simulink model "inverted_pendulum_without_interpreted_function"  (R2018a)
settings: Solver=VariableStepAuto  StartTime=0.0  StopTime=30  RelTol=1e-3
values from neighbouring files (symbols this model uses):
  A = [0 1 0 0 ... (first row only)    [lqr_d_cartpend.m]
  A_d = sys_d.A    [lqr_d_cartpend.m]
  B = [0; 1/M; 0; s*1/(M*L)]    [lqr_d_cartpend.m]
  B_d = sys_d.B    [lqr_d_cartpend.m]
  C = [1 1 1 1]    [lqr_d_cartpend.m]
  C_d = sys_d.C    [lqr_d_cartpend.m]
  Ts = 0.1    [lqr_d_cartpend.m]
  y0 = [-3; 0; pi + pi/4; 0]    [lqr_d_cartpend.m]
undefined symbols (not defined in the file or in its folder): Kd, Obd
libraries: fl_lib x4, nesl_utility x4, elec_lib x3
settings Model: EnablePacing=on  PacingRate=1000  Creator=USER  LastModifiedBy=USER

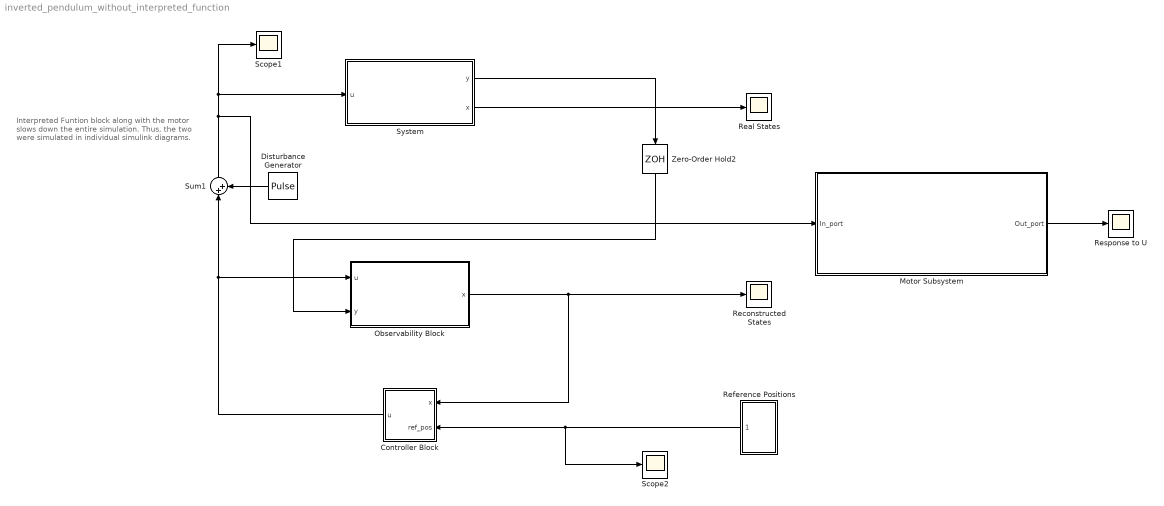
== system inverted_pendulum_without_interpreted_function ==
  note: Interpreted Funtion block along with the motor slows down the entire simulation. Thus, the two were simulated in individual simulink diagrams.
  Controller Block : Subsystem
  Disturbance Generator : DiscretePulseGenerator  PulseType=Time based  Amplitude=20  Period=10  PulseWidth=50  PhaseDelay=10
  Motor Subsystem : Subsystem
  Observability Block : Subsystem
  Real States : Scope
  Reconstructed States : Scope
  Reference Positions : Subsystem
  Response to U : Scope
  Scope1 : Scope
  Scope2 : Scope
  Sum1 : Sum  Inputs=|++
  System : Subsystem
  Zero-Order Hold2 : ZeroOrderHold  SampleTime=Ts
  wires:
  Reference Positions/1(ref_pos) -> Controller Block/2(ref_pos), Scope2/1
  Observability Block/1("x ") -> Reconstructed States/1, Controller Block/1("x ")
  System/1("y ") -> Zero-Order Hold2/1
  Zero-Order Hold2/1 -> Observability Block/2(y)
  System/2("x ") -> Real States/1
  Disturbance Generator/1 -> Sum1/2
  Sum1/1 -> Motor Subsystem/1(In_port), Scope1/1, System/1("u ")
  Motor Subsystem/1(Out_port) -> Response to U/1
  Controller Block/1("u ") -> Sum1/1, Observability Block/1("u ")

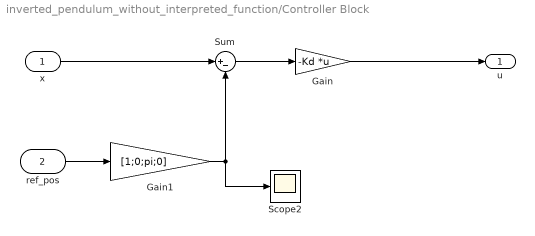
== system inverted_pendulum_without_interpreted_function/Controller Block ==
  "x " : Inport
  ref_pos : Inport  Port=2
  Gain : Gain  Gain=-Kd  Multiplication=Matrix(K*u)
  Gain1 : Gain  Gain=[1;0;pi;0]
  Scope2 : Scope
  Sum : Sum  Inputs=|+-
  "u " : Outport
  wires:
  Gain/1 -> "u "/1
  "x "/1 -> Sum/1
  Sum/1 -> Gain/1
  Gain1/1 -> Scope2/1, Sum/2
  ref_pos/1 -> Gain1/1

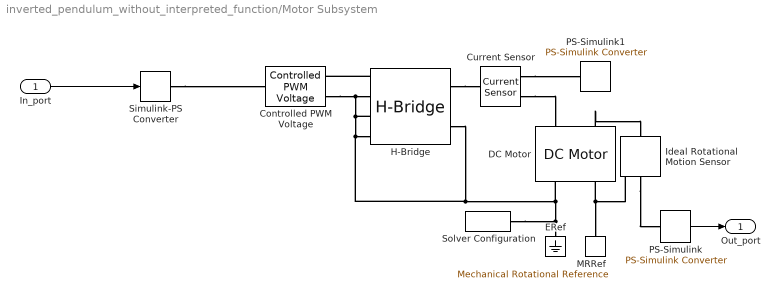
== system inverted_pendulum_without_interpreted_function/Motor Subsystem ==
  In_port : Inport
  Controlled PWM Voltage : elec_lib/Actuators & Drivers/Drivers/Controlled PWM Voltage  F=4000 Hz  TD=0 s  pulse_width_offset=0 s  pulse_min=0 s  Vmin=0 V  Vmax=15 V  Vm=5 V  pwm_or_av=2  event_type=1  sample_time=1e-6 s  u_min=0  u_max=15
      settings: SourceProductName=Simscape Electronics  SourceProductBaseCode=SN
  Current Sensor : fl_lib/Electrical/Electrical Sensors/Current Sensor
      settings: SourceProductName=Foundation Library
  DC Motor : elec_lib/Actuators & Drivers/Rotational Actuators/DC Motor  parameterization=3  Ra=3.38 Ohm  La=0.01 H  emf_or_torque=1  Kv=0.029 V/(rad/s)  Ki=6.876e-04 N*m/A  T_stall=0.1 N*m  w_max=4000 rpm  w_rated=2500 rpm  P_rated=10 W  V_rated=12 V  J=0.0002 kg*m^2  lam_param=1  lam=0.5e-5 N*m/(rad/s)  i_noload=0 A  V_i_noload=1.5 V  speed0=0 rpm  alpha=0.00393 1/K  Tmeas=25 degC  thermal_mass=100 J/K  initial_temperature=25 degC
  ERef : fl_lib/Electrical/Electrical Elements/Electrical Reference
      settings: SourceProductName=Foundation Library
  H-Bridge : elec_lib/Actuators & Drivers/Drivers/H-Bridge  Venable=2.5 V  Vmax=5 V  Vreverse=0.000001 mV  Vbrake=2.5 V  Vm=12 mV  pwm_or_av=2  discontinuous=0  freewheeling_mode=1  freewheeling_mode_disc=1  Ron=0.1 Ohm  Don=0.1 Ohm  Rload=3.38+0.1 Ohm  Lload=1e-5 H  F=4 kHz  thermal_mass=100 J/K  initial_temperature=298.15 K  Ron2=0.1 Ohm  Don2=0.05 Ohm  Tmeas=298.15 K  Tmeas2=398.15 K
      settings: SourceProductName=Simscape Electronics  SourceProductBaseCode=SN
  Ideal Rotational Motion Sensor : fl_lib/Mechanical/Mechanical Sensors/Ideal Rotational Motion Sensor  offset=0 deg
      settings: SourceProductName=Foundation Library
  MRRef : fl_lib/Mechanical/Rotational Elements/Mechanical Rotational Reference
      settings: SourceProductName=Foundation Library
  PS-Simulink : nesl_utility/PS-Simulink Converter  PhysicalDomain=network_engine_domain  SubClassName=ps_output  LeftPortType=input  RightPortType=output  PseudoPeriodic=off  Frequencies=[]  Unit=rpm  AffineConversion=off
  PS-Simulink1 : nesl_utility/PS-Simulink Converter  PhysicalDomain=network_engine_domain  SubClassName=ps_output  LeftPortType=input  RightPortType=output  PseudoPeriodic=off  Frequencies=[]  Unit=A  AffineConversion=off
  Simulink-PS Converter : nesl_utility/Simulink-PS Converter  PhysicalDomain=network_engine_domain  SubClassName=ps_input  LeftPortType=input  RightPortType=output  PseudoPeriodic=off  Frequencies=[]  NoiseDistribution=none  NoiseParameters=[]  Unit=V  AffineConversion=off  FilteringAndDerivatives=provide  SimscapeFilterOrder=1  InputFilterTimeConstant=0.001  UdotUserProvided=0
  Solver Configuration : nesl_utility/Solver Configuration  PhysicalDomain=network_engine_domain  SubClassName=solver  LeftPortType=input  RightPortType=generic  Tones=[]  Harmonics=[]  SimulateNoise=off  Profile=off  UseLocalSampling=off  EnableSwitchedLinearOptims=on  FrequencyDomain=off  UseCCode=off  RelTol=0.001  AbsTol=1e-06  MinStep=1e-09  ToWorkspace=off  RevertToSquareIcSolve=off  NumHomotopyIterations=100  PhasorMode=off  PhasorModeNumHarmonics=1  DoDC=off  ResidualTolerance=1e-9  UseLocalSolver=off  LocalSolverChoice=NE_BACKWARD_EULER_ADVANCER  LocalSolverSampleTime=.001  DoFixedCost=off  MaxNonlinIter=3  MaxModeIter=2  LinearAlgebra=Sparse  EquationFormulation=NE_TIME_EF  DelaysMemoryBudget=1024  AutomaticFiltering=on  FilteringTimeConstant=0.001
  Out_port : Outport
  wires:
  PS-Simulink/1 -> Out_port/1
  In_port/1 -> Simulink-PS Converter/1
  connections:
  Ideal Rotational Motion Sensor/RConn1 -- DC Motor/RConn2 -- MRRef/LConn1
  H-Bridge/LConn1 -- Controlled PWM Voltage/RConn1
  Simulink-PS Converter/RConn1 -- Controlled PWM Voltage/LConn1
  DC Motor/LConn2 -- Ideal Rotational Motion Sensor/LConn1
  Current Sensor/RConn1 -- PS-Simulink1/LConn1
  Current Sensor/RConn2 -- DC Motor/LConn1
  Ideal Rotational Motion Sensor/RConn2 -- PS-Simulink/LConn1
  H-Bridge/RConn1 -- Current Sensor/LConn1
  ERef/LConn1 -- Solver Configuration/RConn1 -- H-Bridge/LConn3 -- Controlled PWM Voltage/RConn2 -- H-Bridge/LConn2 -- H-Bridge/LConn4 -- H-Bridge/RConn2 -- DC Motor/RConn1

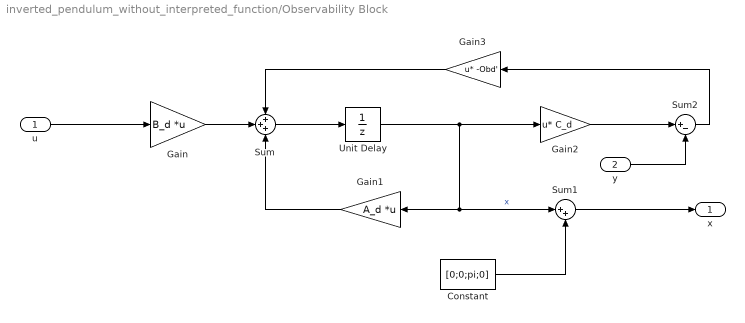
== system inverted_pendulum_without_interpreted_function/Observability Block ==
  "u " : Inport
  y : Inport  Port=2
  Constant : Constant  Value=[0;0;pi;0]
  Gain : Gain  Gain=B_d  Multiplication=Matrix(K*u)
  Gain1 : Gain  Gain=A_d  Multiplication=Matrix(K*u) (u vector)
  Gain2 : Gain  Gain=C_d  Multiplication=Matrix(u*K)
  Gain3 : Gain  Gain=-Obd'  Multiplication=Matrix(u*K)
  Sum : Sum  Inputs=+++
  Sum1 : Sum  Inputs=|++
  Sum2 : Sum  Inputs=|+-
  Unit Delay : UnitDelay  InitialCondition=y0*0  SampleTime=Ts
  "x " : Outport
  wires:
  Sum/1 -> Unit Delay/1
  "u "/1 -> Gain/1
  Gain/1 -> Sum/2
  Unit Delay/1 -> Sum1/1, Gain1/1, Gain2/1  "x"
  Sum1/1 -> "x "/1
  Constant/1 -> Sum1/2
  Gain2/1 -> Sum2/1
  y/1 -> Sum2/2
  Sum2/1 -> Gain3/1
  Gain1/1 -> Sum/3
  Gain3/1 -> Sum/1

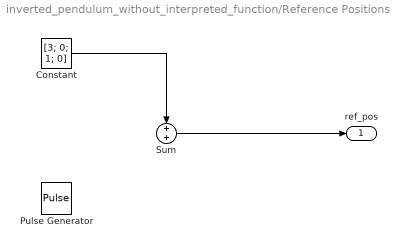
== system inverted_pendulum_without_interpreted_function/Reference Positions ==
  Constant : Constant  Value=[3; 0; 1; 0]
  Pulse Generator : DiscretePulseGenerator  PulseType=Time based  Amplitude=[2;0.3;0;-0.5]  Period=14  PulseWidth=50  PhaseDelay=10
  Sum : Sum
  ref_pos : Outport
  wires:
  Sum/1 -> ref_pos/1
  Constant/1 -> Sum/1

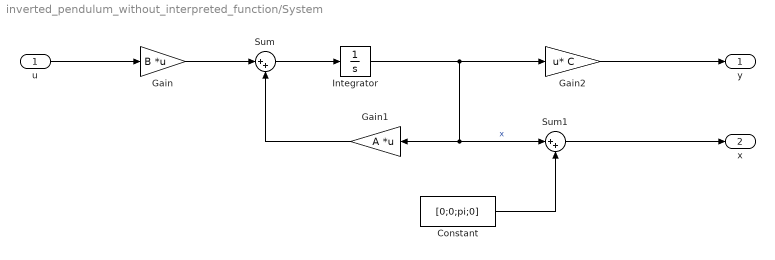
== system inverted_pendulum_without_interpreted_function/System ==
  "u " : Inport
  Constant : Constant  Value=[0;0;pi;0]
  Gain : Gain  Gain=B  Multiplication=Matrix(K*u)
  Gain1 : Gain  Gain=A  Multiplication=Matrix(K*u) (u vector)
  Gain2 : Gain  Gain=C  Multiplication=Matrix(u*K)
  Integrator : Integrator  InitialCondition=[-3; -0.3; pi/10*4; 0.5]
  Sum : Sum  Inputs=|++
  Sum1 : Sum  Inputs=|++
  "y " : Outport
  "x " : Outport  Port=2
  wires:
  Sum/1 -> Integrator/1
  "u "/1 -> Gain/1
  Gain/1 -> Sum/1
  Gain1/1 -> Sum/2
  Gain2/1 -> "y "/1
  Integrator/1 -> Gain2/1, Sum1/1, Gain1/1  "x"
  Sum1/1 -> "x "/1
  Constant/1 -> Sum1/2
